simulink model "mengpH_m"  (Simulink 8.5)
settings: Solver=ode45  SolverMode=SingleTasking  StartTime=0.0  StopTime=999999  MaxStep=10  RelTol=1e-3  AbsTol=1e-3
values from neighbouring files (symbols this model uses):
  U = st_Varia('LongNames')    [mengpH_i.m]
  x0 = []    [mengpH_i.m]    (also in mengpH_s.m = x0)
undefined symbols (not defined in the file or in its folder): B
settings Model: Creator=M.Sparnaaij  LastModifiedBy=Martijn
settings DataIOCC: LimitDataPoints=off  SaveOutput=off  SaveTime=off  SignalLoggingName=sigsOut
settings OptimizationCC: BooleanDataType=off
settings DebuggingCC: SaveWithParameterizedLinksMsg=none  SignalResolutionControl=TryResolveAllWithWarning  MultiTaskDSMMsg=warning  MultiTaskCondExecSysMsg=none  FcnCallInpInsideContextMsg=EnableAllAsWarning  StrictBusMsg=None
settings HardwareCC: TargetUnknown=on

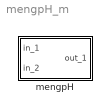
== system mengpH_m ==
  mengpH : Subsystem  Description=mengpH
      mask init:
      | filenaam='.\StimelaData\mengpH_p.mat';
      | 
      | [Pn,Fn,Fext]=Fileprop(filenaam);
      | 
      | errstr = st_UniqName(filenaam,'filenaam=''','SubSystem','OpenFcn');
      | if errstr, error([errstr 'The filename "' filenaam '" is already in use. Choose a different filename.']), end
      | 
      | P = mengpH_p(filenaam);
      | [B,x0,U]=mengpH_i(filenaam);
      | V = st_Varia;
      settings: OpenFcn=|
      | filenaam='.\StimelaData\mengpH_p.mat';
      | st_ParameterInput('init',gcb,filenaam,'mengpH');
      mask Display:
      | plot(0,0,100,100,[0 20],[85 85],[0 20],[80 80],[0 20],[20 20],[0 20],[15 15],[80 100],[ 50 50],[80 100],[ 55 55],[20 80 80 20 20],[10 10 90  90 10]);
      | disp('')
      | text(50,50,'mengpH', 'horizontalAlignment', 'center', 'verticalAlignment', 'middle');
      | text(50,0,Fn, 'horizontalAlignment', 'center', 'verticalAlignment', 'base');

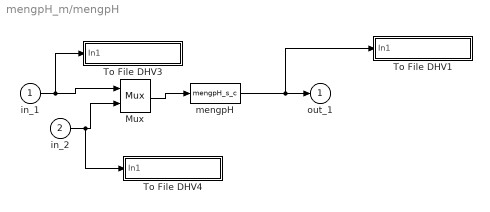
== system mengpH_m/mengpH ==
  in_1 : Inport
  in_2 : Inport  Port=2
  Mux : Mux  Inputs=[U.Number B.Setpoints]
  To File DHV1 : Subsystem  mask(To File DHV){naam=[filenaam(1:length(filenaam)-4) '_out.sti']}
      mask prompts: naam "Naam van bestand"
      mask init:
      | set_param([gcb '/To File'],'Filename',naam);
      mask Display: disp(naam)
  To File DHV3 : Subsystem  mask(To File DHV){naam=[filenaam(1:length(filenaam)-4) '_in.sti']}
      mask prompts: naam "Naam van bestand"
      mask init:
      | set_param([gcb '/To File'],'Filename',naam);
      mask Display: disp(naam)
  To File DHV4 : Subsystem  mask(To File DHV){naam=[filenaam(1:length(filenaam)-4) '_ES.sti']}
      mask prompts: naam "Naam van bestand"
      mask init:
      | set_param([gcb '/To File'],'Filename',naam);
      mask Display: disp(naam)
  mengpH : S-Function  FunctionName=mengpH_s_c  Parameters=B,x0,U,P
  out_1 : Outport  InitialOutput=0
  wires:
  in_2/1 -> To File DHV4/1(In1), Mux/2
  in_1/1 -> To File DHV3/1(In1), Mux/1
  Mux/1 -> mengpH/1
  mengpH/1 -> To File DHV1/1(In1), out_1/1

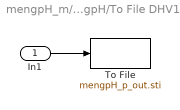
== system mengpH_m/mengpH/To File DHV1 ==
  In1 : Inport
  To File : ToFile  Filename=mengpH_p_out.sti  MatrixName=mengpHout
  wires:
  In1/1 -> To File/1

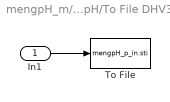
== system mengpH_m/mengpH/To File DHV3 ==
  In1 : Inport
  To File : ToFile  Filename=mengpH_p_in.sti  MatrixName=mengpHin
  wires:
  In1/1 -> To File/1

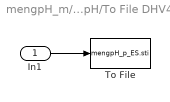
== system mengpH_m/mengpH/To File DHV4 ==
  In1 : Inport
  To File : ToFile  Filename=mengpH_p_ES.sti  MatrixName=mengpHES
  wires:
  In1/1 -> To File/1
